simulink model "PMSM_PI_decomposition_workin2"  (R2024a)
settings: Solver=VariableStepAuto  StartTime=0.0  StopTime=10  FixedStep=0.000025  MinStep=0.000002  RelTol=1e-4  EnableMultiTasking=on
InitFcn:
  | Ts = 10e-6;
  | 
  | R = 0.958;
  | Ld = 5.25e-3;
  | Lq = 12e-3;
  | Pn = 4;
  | flux = 0.1827;
values from neighbouring files (symbols this model uses):
  Flux = 0.1827    [Parameters.m]    (also in StateSpace.m = 0.192)
  Kid = Kpd*(Rs/Ld)    (= 157.079632679)    [StateSpace.m]
  Kiq = Kpd*(Rs/Lq)    (= 157.079632679)    [StateSpace.m]
  Kpd = (Ld*2*pi*fsw)/10    (= 2.4975661596)    [StateSpace.m]
  Kpq = (Lq*2*pi*fsw)/10    (= 2.4975661596)    [StateSpace.m]
  L_d = 0.00525    [Parameters.m]
  L_q = 0.00525    [Parameters.m]
  p = 4    [Parameters.m]    (also in StateSpace.m)
  R_s = 0.9585    [Parameters.m]
  vdc = 560    [StateSpace.m]
libraries: mcbcontrolslib x4, spsControlledVoltageSourceLib x2, spsDCVoltageSourceLib x1, mcbhdlpositiondecoderlib x1, mcbpmsmnonlinearlib x1, spsPermanentMagnetSynchronousMachineLib x1, spsSVPWMGenerator2LevelLib x1, simulink x1, spsUniversalBridgeLib x1, sps_lib x1
settings Model: Creator=SUN  LastModifiedBy=didad
settings SolverCC: InitialStep=0.000002  ZeroCrossControl=DisableAll  AlgebraicLoopSolver=TrustRegion
settings DataIOCC: LimitDataPoints=on  SaveFormat=Array  SignalLoggingSaveFormat=ModelDataLogs  ReturnWorkspaceOutputs=off
settings OptimizationCC: ExpressionDepthLimit=2147483647  InitFltsAndDblsToZero=on  LifeSpan=inf
settings DebuggingCC: UnderspecifiedInitializationDetection=Classic  MergeDetectMultiDrivingBlocksExec=none  SolverPrmCheckMsg=warning  FcnCallInpInsideContextMsg=warning  UnconnectedInputMsg=warning  UnconnectedOutputMsg=warning  UnconnectedLineMsg=warning  StateNameClashWarn=warning  SFUnexpectedBacktrackingDiag=warning  SFNoUnconditionalDefaultTransitionDiag=warning  SFExecutionAtInitializationDiag=none  ArithmeticOperatorsInVariantConditions=warning
settings HardwareCC: ProdBitPerPointer=32  ProdBitPerSizeT=32  ProdBitPerPtrDiffT=32  ProdLargestAtomicFloat=None  ProdIntDivRoundTo=Undefined  ProdEndianess=Unspecified  ProdWordSize=32  ProdHWDeviceType=32-bit Generic
settings ModelReferenceCC: EnableRefExpFcnMdlSchedulingChecks=on  PropagateSignalLabelsOutOfModel=off
settings SFSimCC: SimUseLocalCustomCode=off  CustomCodeUndefinedFunction=UseInterfaceOnly
settings RTWCC: RTWUseLocalCustomCode=off  GPUComputeCapability=3.5
settings CodeAppCC: StateflowObjectComments=on
settings GRTTargetCC: TargetLangStandard=C89/C90 (ANSI)  CombineOutputUpdateFcns=off  GRTInterface=on
settings ConfigComp: CovMetricSettings=dw  CovSaveCumulativeToWorkspaceVar=on  CovSaveSingleToWorkspaceVar=on  CovExternalEMLEnable=off  CovSFcnEnable=off
settings SimscapeCC: SimscapeNormalizeSystem=off

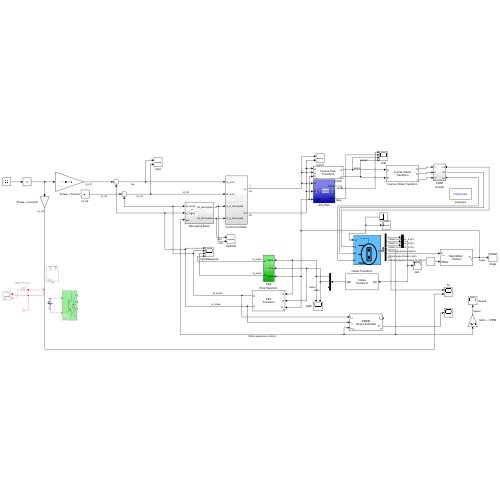
[thumbnail: Simulink's stored preview of the top-level diagram]
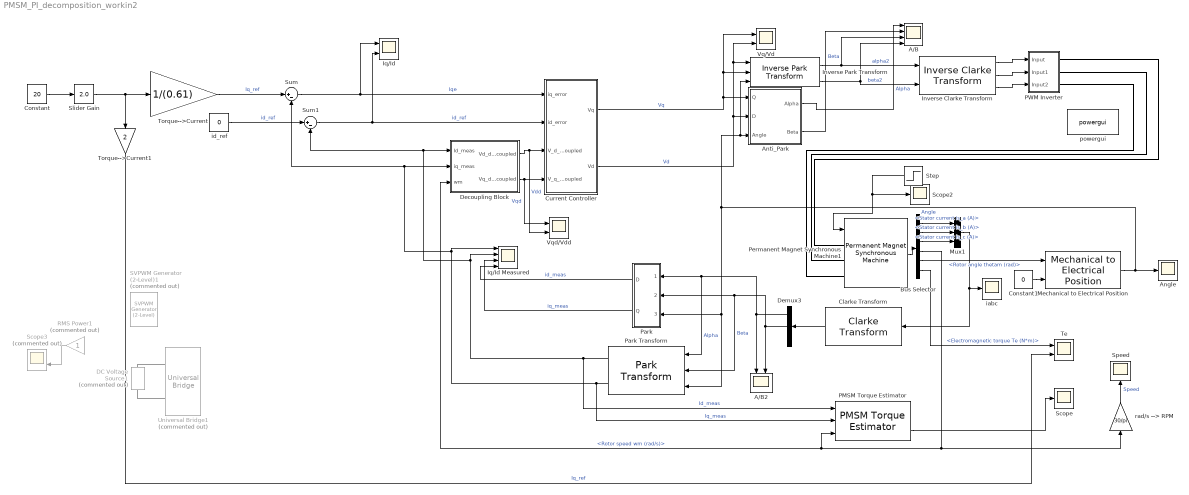
== system PMSM_PI_decomposition_workin2 ==
  A/B : Scope  NumInputPorts=4
  A/B2 : Scope  NumInputPorts=2
  Angle : Scope
  Anti_Park : Subsystem
  Bus Selector : BusSelector  OutputSignals=Stator current is_a (A),Stator current is_b (A),Stator current is_c (A),Rotor speed wm (rad/s),Rotor angle thetam (rad),Electromagnetic torque Te (N*m)
  Clarke Transform : mcbcontrolslib/Clarke Transform  VariantControl=Variant2  PhaseInput=Three inputs  EnPowerInv=off
      settings: LibrarySourceBlock=mcblib/Controls/Math Transforms/Clarke Transform
  Constant : Constant  Value=20
  Constant1 : Constant  Value=0
  Current Controller : Subsystem
  DC Voltage Source1 : spsDCVoltageSourceLib/DC Voltage Source  Commented=on  Amplitude=vdc  Measurements=None
  Decoupling Block : Subsystem
  Demux3 : Demux  Outputs=3
  Inverse Clarke Transform : mcbcontrolslib/Inverse Clarke Transform  PhaseInput=Two inputs  EnPowerInv=off
      settings: LibrarySourceBlock=mcbhdllib/Controls/Math Transforms/Inverse Clarke Transform
  Inverse Park Transform : mcbcontrolslib/Inverse Park Transform  PhaseInput=Two inputs  AxisAlignment=D-axis  ThetaInput=Electrical position  AngleInput=Radians  N_points=1024
      settings: LibrarySourceBlock=mcbhdllib/Controls/Math Transforms/Inverse Park Transform
  Iq/Id : Scope  NumInputPorts=2
  Iq/Id Measured : Scope  NumInputPorts=4
  Mechanical to Electrical Position : mcbhdlpositiondecoderlib/Mechanical to Electrical Position  PolePairsInputType=Specify via dialog  NrPP=p  selectedRange=Radians  MechOfstInputType=Input port  mechOffsetIn=0  maxAngleIn=2*pi  InputDataType=single  VariantSelect=floating-point
      settings: LibrarySourceBlock=mcbhdllib/Sensor Decoders/Mechanical to Electrical Position
  Mux1 : Mux  Inputs=3
  PMSM Torque Estimator : mcbpmsmnonlinearlib/PMSM Torque Estimator  polePairs=4  nonLinearityChoice=Linear model with lumped parameters  Ld=L_d  Lq=L_q  FluxPM=Flux  idVec=[-40, -20, 0, 20]  iqVec=[-40, -20, 0, 20, 40]  LdTable=0.2e-3 * ones(4, 5)  LqTable=0.2e-3 * ones(4, 5)  FluxPMTable=6.4e-3 * ones(4, 5)  FluxDTable=[-1.6,-1.6,-1.6,-1.6,-1.6;2.4,2.4,2.4,2.4,2.4;6.4,6.4,6.4,6.4,6.4;10.4,10.4,10.4,10.4,10.4]*1e-3  FluxQTable=[-8,-4,0,4,8;-8,-4,0,4,8;-8,-4,0,4,8;-8,-4,0,4,8]*1e-3  Units=Per-Unit (PU)  V_base=24/sqrt(3)  I_base=19.3  N_base=4107  T_base=22.2336  P_base=401.143  scaledTables=on
      settings: LibrarySourceBlock=mcblib/Controls/Control Reference/PMSM Torque Estimator
  PWM Inverter : Subsystem
  Park : Subsystem
  Park Transform : mcbcontrolslib/Park Transform  PhaseInput=Two inputs  AxisAlignment=D-axis  ThetaInput=Electrical position  AngleInput=Radians  N_points=1024
      settings: LibrarySourceBlock=mcblib/Controls/Math Transforms/Park Transform
  Permanent Magnet Synchronous Machine1 : spsPermanentMagnetSynchronousMachineLib/Permanent Magnet Synchronous Machine  NbPhases=3  FluxDistribution=Sinusoidal  RotorType=Round  MechanicalLoad=Speed w  PresetModel="15:  87.75 Nm 560 Vdc 3000 RPM - 97.96 Nm"  ShowDetailedParameters=on  MeasurementBus=off  Resistance=0.05  Inductance=8.5e-3  dqInductances=[5.25e-3,12e-3]  La=0.000795  MachineConstant=Flux linkage established by magnets (V.s)  Flux=0.192  VoltageCst=139.2998  TorqueCst=1.152  Flat=120  Mechanical=[0.011 0.001417 4 0]  PolePairs=4  InitialConditions=[0,0, 0,0]  InitialConditions5ph=[0 0 0 0 0 0]  RefAngle=Aligned with phase A axis (original Park)  IterativeDiscreteModel=Trapezoidal non iterative  TsBlock=-1  TsPowergui=0
  RMS Power1 : Gain  Commented=on
  SVPWM Generator (2-Level)1 : spsSVPWMGenerator2LevelLib/SVPWM Generator (2-Level)  Commented=on  InputType=alpha-beta components  SwitchingPattern=Pattern #1  Fc=fsw  ParUref=[0.8 -30 50]  Ts=0
  Scope : Scope
  Scope2 : Scope
  Scope3 : Scope  Commented=on  NumInputPorts=2
  Slider Gain : simulink/Math Operations/Slider Gain  gain=2.0  low=0  high=2
  Speed : Scope
  Step : Step  Time=0.1  After=0.2  SampleTime=0
  Sum : Sum  Inputs=|+-
  Sum1 : Sum  Inputs=|+-
  Te : Scope  NumInputPorts=2
  Torque-->Current : Gain  Gain=1/(0.61)
  Torque-->Current1 : Gain  Gain=2
  Universal Bridge1 : spsUniversalBridgeLib/Universal Bridge  Commented=on  Arms=3  SnubberResistance=1e-5  SnubberCapacitance=inf  Device=IGBT / Diodes  Ron=1e-3  Lon=0  ForwardVoltages="[  0  0  ]"  ForwardVoltage=0  GTOparameters=[ 10e-6 , 20e-6 ]  IGBTparameters=[ 1e-6 , 2e-6 ]  Measurements=None  Measurements_2=None  converterType=Rectifier
  Vq/Vd : Scope  NumInputPorts=2
  Vqd/Vdd : Scope  NumInputPorts=2
  iabc : Scope
  id_ref : Constant  Value=0
  powergui : sps_lib/powergui  Priority=1  SimulationMode=Continuous  SampleTime=50e-6  frequency=60  Iterations=50  frequencyindice=0  Pbase=100e6  ErrMax=1e-4  UnitsV=kV  UnitsW=MW  buscounter=0  FunctionMessages=off  echomessages=off  EnableUseOfTLC=off  CurrentSourceSwitches=off  DisableSnubberDevices=off  DisableRonSwitches=off  DisableVfSwitches=off  DisplayEquations=off  AutomaticDiscreteSolvers=off  SolverType=Tustin/Backward Euler (TBE)  Interpol=off  ExternalGateDelay=off  methode=off  Ts=100  x0status=blocks  SPID=on  SwTol=0  HookPort=off  NonlinearTolerance=1e-4  nMaxIteration=100  ContinueOnMaxIteration=off  RestoreLinks=warning  ResistiveCurrentMeasurement=off  Frange=[0:2:500]  Ylog=off  Xlog=on  ShowGrid=off  save=off  variable=ZData  structure=0  ZoomFFT=off  StartTime=0.0  cycles=1  DisplayStyle=1  fundamental=60  FreqAxis=off  MaxFrequency=1000  frequencyindicesteady=1  RmsSteady=1  display=off
  rad/s --> RPM : Gain  Gain=30/pi
  wires:
  Step/1 -> Permanent Magnet Synchronous Machine1/1, Scope2/1
  Bus Selector/3 -> Mux1/3  "<Stator current is_c (A)>"
  Bus Selector/2 -> Mux1/2  "<Stator current is_b (A)>"
  Bus Selector/1 -> Mux1/1  "<Stator current is_a (A)>"
  Permanent Magnet Synchronous Machine1/1 -> Bus Selector/1
  id_ref/1 -> Sum1/1  "id_ref"
  Sum/1 -> Current Controller/1(iq_error), Iq/Id/1  "Iqe"
  Park Transform/2 -> PMSM Torque Estimator/2, Sum/2, Decoupling Block/2(iq_meas), Iq/Id Measured/1  "Iq_meas"
  Slider Gain/1 -> Torque-->Current1/1, Torque-->Current/1
  Park Transform/1 -> PMSM Torque Estimator/1, Iq/Id Measured/2, Sum1/2, Decoupling Block/1(Id_meas)  "Id_meas"
  Bus Selector/4 -> PMSM Torque Estimator/3, Decoupling Block/3(wm), rad/s --> RPM/1  "<Rotor speed wm (rad/s)>"
  Mux1/1 -> Clarke Transform/1, iabc/1
  rad/s --> RPM/1 -> Speed/1  "Speed"
  Demux3/1 -> A/B2/1, Park Transform/1, Park/1(Alpha)  "Alpha"
  Demux3/2 -> A/B2/2, Park Transform/2, Park/2(Beta)  "Beta"
  Bus Selector/5 -> Mechanical to Electrical Position/1  "<Rotor angle thetam (rad)>"
  Mechanical to Electrical Position/1 -> Park Transform/3, Park/3(Angle), Inverse Park Transform/3, Anti_Park/3(Angle), Angle/1  "Angle"
  Constant1/1 -> Mechanical to Electrical Position/2
  Decoupling Block/1(Vd_decoupled) -> Current Controller/3(V_d_decoupled), Vqd/Vdd/2  "Vdd"
  Decoupling Block/2(Vq_decoupled) -> Current Controller/4(V_q_decoupled), Vqd/Vdd/1  "Vqd"
  Constant/1 -> Slider Gain/1
  Current Controller/2(Vd) -> Inverse Park Transform/1, Vq/Vd/2, Anti_Park/2(D)  "Vd"
  Current Controller/1(Vq) -> Inverse Park Transform/2, Vq/Vd/1, Anti_Park/1(Q)  "Vq"
  Clarke Transform/1 -> Demux3/1
  Inverse Park Transform/1 -> A/B/3, Inverse Clarke Transform/1  "alpha2"
  Inverse Park Transform/2 -> A/B/4, Inverse Clarke Transform/2  "beta2"
  Anti_Park/1(Alpha) -> A/B/1  "Alpha"
  Anti_Park/2(Beta) -> A/B/2  "Beta"
  Park/1(D) -> Iq/Id Measured/4  "id_meas"
  Park/2(Q) -> Iq/Id Measured/3  "iq_meas"
  Torque-->Current/1 -> Sum/1  "Iq_ref"
  Bus Selector/6 -> Te/1  "<Electromagnetic torque Te (N*m)>"
  PMSM Torque Estimator/2 -> Scope/1
  ? -> Scope3/1
  ? -> RMS Power1/1
  RMS Power1/1 -> Scope3/2
  Inverse Clarke Transform/1 -> PWM Inverter/1(Input)
  Inverse Clarke Transform/2 -> PWM Inverter/2(Input1)
  Inverse Clarke Transform/3 -> PWM Inverter/3(Input2)
  Sum1/1 -> Iq/Id/2, Current Controller/2(id_error)  "id_ref"
  Torque-->Current1/1 -> Te/2  "Iq_ref"
  connections:
  Universal Bridge1/RConn1 -- DC Voltage Source1/RConn1
  DC Voltage Source1/LConn1 -- Universal Bridge1/RConn2
  PWM Inverter/RConn1 -- Permanent Magnet Synchronous Machine1/LConn1
  PWM Inverter/RConn2 -- Permanent Magnet Synchronous Machine1/LConn2
  PWM Inverter/RConn3 -- Permanent Magnet Synchronous Machine1/LConn3

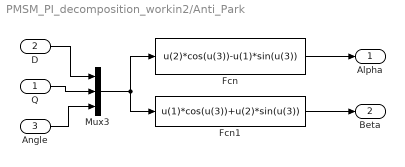
== system PMSM_PI_decomposition_workin2/Anti_Park ==
  Q : Inport
  D : Inport  Port=2
  Angle : Inport  Port=3
  Fcn : Fcn  Expr=u(2)*cos(u(3))-u(1)*sin(u(3))
  Fcn1 : Fcn  Expr=u(1)*cos(u(3))+u(2)*sin(u(3))
  Mux3 : Mux  Inputs=3
  Alpha : Outport  VectorParamsAs1DForOutWhenUnconnected=off
  Beta : Outport  Port=2  VectorParamsAs1DForOutWhenUnconnected=off
  wires:
  Angle/1 -> Mux3/3
  Fcn1/1 -> Beta/1
  Mux3/1 -> Fcn1/1, Fcn/1
  Fcn/1 -> Alpha/1
  D/1 -> Mux3/1
  Q/1 -> Mux3/2

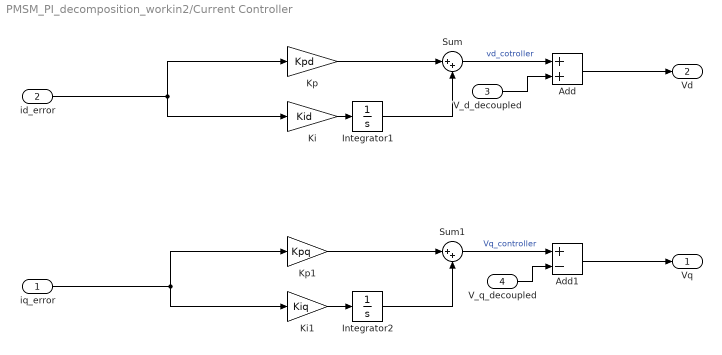
== system PMSM_PI_decomposition_workin2/Current Controller ==
  iq_error : Inport
  id_error : Inport  Port=2
  V_d_decoupled : Inport  Port=3
  V_q_decoupled : Inport  Port=4
  Add : Sum
  Add1 : Sum  Inputs=+-
  Integrator1 : Integrator
  Integrator2 : Integrator
  Ki : Gain  Gain=Kid
  Ki1 : Gain  Gain=Kiq
  Kp : Gain  Gain=Kpd
  Kp1 : Gain  Gain=Kpq
  Sum : Sum  Inputs=|++
  Sum1 : Sum  Inputs=|++
  Vq : Outport
  Vd : Outport  Port=2
  wires:
  V_q_decoupled/1 -> Add1/2
  Ki1/1 -> Integrator2/1
  V_d_decoupled/1 -> Add/2
  Kp1/1 -> Sum1/1
  Integrator2/1 -> Sum1/2
  Integrator1/1 -> Sum/2
  Ki/1 -> Integrator1/1
  Kp/1 -> Sum/1
  Sum/1 -> Add/1  "vd_cotroller"
  Sum1/1 -> Add1/1  "Vq_controller"
  Add/1 -> Vd/1
  Add1/1 -> Vq/1
  id_error/1 -> Ki/1, Kp/1
  iq_error/1 -> Ki1/1, Kp1/1

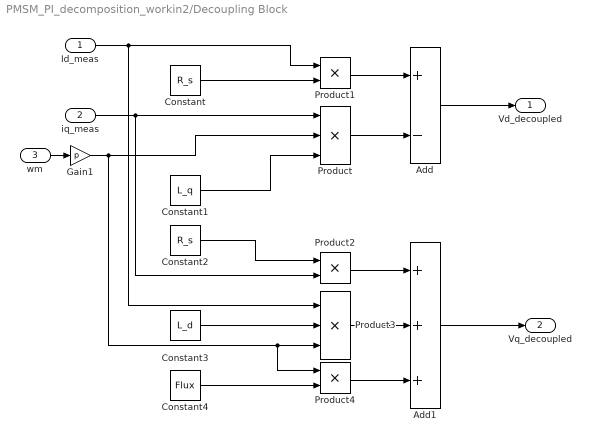
== system PMSM_PI_decomposition_workin2/Decoupling Block ==
  Id_meas : Inport
  iq_meas : Inport  Port=2
  wm : Inport  Port=3
  Add : Sum  Inputs=+-
  Add1 : Sum  Inputs=+++
  Constant : Constant  Value=R_s
  Constant1 : Constant  Value=L_q
  Constant2 : Constant  Value=R_s
  Constant3 : Constant  Value=L_d
  Constant4 : Constant  Value=Flux
  Gain1 : Gain  Gain=p
  Product : Product  Inputs=3
  Product1 : Product
  Product2 : Product
  Product3 : Product  Inputs=3
  Product4 : Product
  Vd_decoupled : Outport
  Vq_decoupled : Outport  Port=2
  wires:
  Add/1 -> Vd_decoupled/1
  Product1/1 -> Add/1
  Constant/1 -> Product1/2
  Id_meas/1 -> Product1/1, Product3/1
  Product/1 -> Add/2
  Gain1/1 -> Product4/1, Product3/3, Product/2
  Constant1/1 -> Product/3
  Add1/1 -> Vq_decoupled/1
  Product2/1 -> Add1/1
  Constant2/1 -> Product2/1
  iq_meas/1 -> Product/1, Product2/2
  Product3/1 -> Add1/2
  Constant3/1 -> Product3/2
  Product4/1 -> Add1/3
  Constant4/1 -> Product4/2
  wm/1 -> Gain1/1

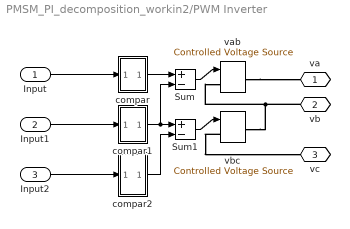
== system PMSM_PI_decomposition_workin2/PWM Inverter ==
  Input : Inport
  Input1 : Inport  Port=2
  Input2 : Inport  Port=3
  Sum : Sum  Inputs=+-  InputSameDT=on  SaturateOnIntegerOverflow=on  OutDataTypeStr=Inherit: Same as first input
  Sum1 : Sum  Inputs=+-  InputSameDT=on  SaturateOnIntegerOverflow=on  OutDataTypeStr=Inherit: Same as first input
  compar : Subsystem
  compar1 : Subsystem
  compar2 : Subsystem
  vab : spsControlledVoltageSourceLib/Controlled Voltage Source  Description=source block  Initialize=on  Source_Type=AC  Amplitude=0  Phase=0  Frequency=0  Measurements=None
      settings: AttributesFormatString=\n
  vbc : spsControlledVoltageSourceLib/Controlled Voltage Source  Description=source block  Initialize=on  Source_Type=AC  Amplitude=0  Phase=0  Frequency=0  Measurements=None
      settings: AttributesFormatString=\n
  va : PMIOPort  Side=Right
  vb : PMIOPort  Port=2  Side=Right
  vc : PMIOPort  Port=3  Side=Right
  wires:
  compar/1(va) -> Sum/1
  compar1/1(vb) -> Sum/2, Sum1/1
  compar2/1(vc) -> Sum1/2
  Sum/1 -> vab/1
  Sum1/1 -> vbc/1
  Input/1 -> compar/1(ia)
  Input1/1 -> compar1/1(ib)
  Input2/1 -> compar2/1(ic)
  connections:
  vab/RConn1 -- va/RConn1
  vb/RConn1 -- vab/LConn1 -- vbc/RConn1
  vbc/LConn1 -- vc/RConn1

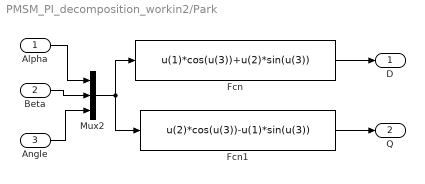
== system PMSM_PI_decomposition_workin2/Park ==
  Alpha : Inport
  Beta : Inport  Port=2
  Angle : Inport  Port=3
  Fcn : Fcn  Expr=u(1)*cos(u(3))+u(2)*sin(u(3))
  Fcn1 : Fcn  Expr=u(2)*cos(u(3))-u(1)*sin(u(3))
  Mux2 : Mux  Inputs=3
  D : Outport  VectorParamsAs1DForOutWhenUnconnected=off
  Q : Outport  Port=2  VectorParamsAs1DForOutWhenUnconnected=off
  wires:
  Beta/1 -> Mux2/2
  Mux2/1 -> Fcn1/1, Fcn/1
  Angle/1 -> Mux2/3
  Alpha/1 -> Mux2/1
  Fcn1/1 -> Q/1
  Fcn/1 -> D/1

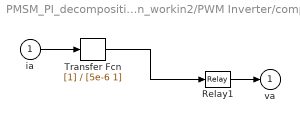
== system PMSM_PI_decomposition_workin2/PWM Inverter/compar ==
  ia : Inport
  Relay1 : Relay  OnSwitchValue=0.05  OffSwitchValue=-0.05  OnOutputValue=155  OffOutputValue=-155
  Transfer Fcn : TransferFcn  Denominator=[5e-6 1]
  va : Outport  InitialOutput=0  VectorParamsAs1DForOutWhenUnconnected=off
  wires:
  Transfer Fcn/1 -> Relay1/1
  Relay1/1 -> va/1
  ia/1 -> Transfer Fcn/1

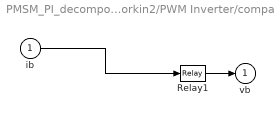
== system PMSM_PI_decomposition_workin2/PWM Inverter/compar1 ==
  ib : Inport
  Relay1 : Relay  OnSwitchValue=0.05  OffSwitchValue=-0.05  OnOutputValue=155  OffOutputValue=-155
  vb : Outport  InitialOutput=0  VectorParamsAs1DForOutWhenUnconnected=off
  wires:
  ib/1 -> Relay1/1
  Relay1/1 -> vb/1

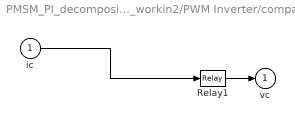
== system PMSM_PI_decomposition_workin2/PWM Inverter/compar2 ==
  ic : Inport
  Relay1 : Relay  OnSwitchValue=0.05  OffSwitchValue=-0.05  OnOutputValue=155  OffOutputValue=-155
  vc : Outport  InitialOutput=0  VectorParamsAs1DForOutWhenUnconnected=off
  wires:
  ic/1 -> Relay1/1
  Relay1/1 -> vc/1
